simulink model "smd_open"  (R2025a)
settings: Solver=ode45  StartTime=0.0  StopTime=15  RelTol=1e-3
settings Model: Creator=rexwang  LastModifiedBy=rexwang

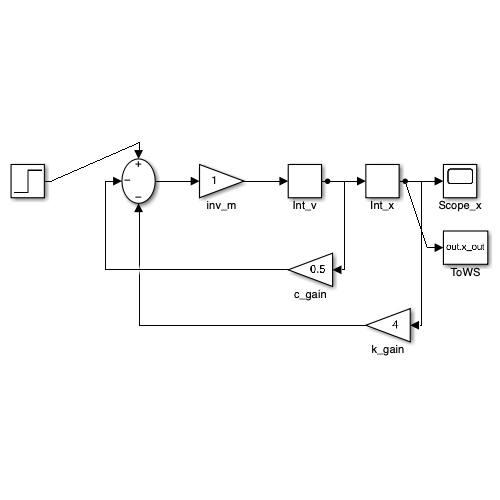
[thumbnail: Simulink's stored preview of the top-level diagram]
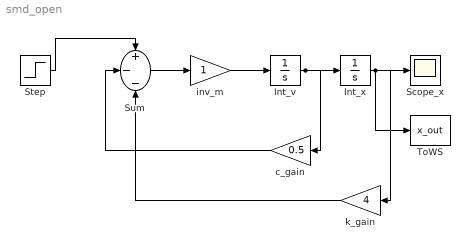
== system smd_open ==
  Int_v : Integrator
  Int_x : Integrator
  Scope_x : Scope
  Step : Step  Time=0  SampleTime=0
  Sum : Sum  Inputs=+--
  ToWS : ToWorkspace  VariableName=x_out  SaveFormat=Structure With Time  SampleTime=-1
  c_gain : Gain  Gain=0.5
  inv_m : Gain
  k_gain : Gain  Gain=4
  wires:
  Step/1 -> Sum/1
  Sum/1 -> inv_m/1
  inv_m/1 -> Int_v/1
  Int_v/1 -> Int_x/1, c_gain/1
  Int_x/1 -> Scope_x/1, ToWS/1, k_gain/1
  c_gain/1 -> Sum/2
  k_gain/1 -> Sum/3
